simulink model "LSM_with_Simulek_CLM"  (R2016a)
settings: Solver=VariableStepAuto  StartTime=0.0  StopTime=2  RelTol=1e-3
values from neighbouring files (symbols this model uses):
  Theta = inv(R'*R)*R'*Y    [LSM with n=0 _ 1_1023 + 1105.m]    (also in LSM with n=2 _ more_1105.m = inv(R'*R)*R'* (Y2'); LSM_with_Simulek_1218.m = inv(X2'*X2)*X2'*Fs)
  Theta_c = inv(X2'*X2)*X2'*Fs    [Constrained_Least_Square_Method_CLM_1218.m]
undefined symbols (not defined in the file or in its folder): g, ks, kv, m
libraries: simulink x1
settings Model: Creator=lg079127  LastModifiedBy=lg079127

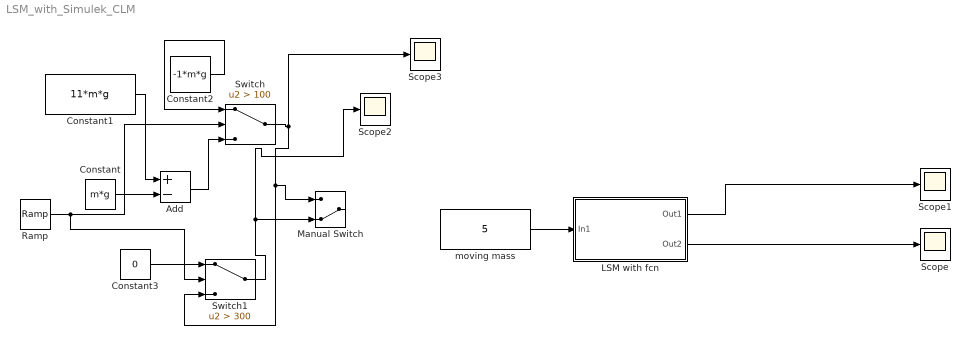
== system LSM_with_Simulek_CLM ==
  Add : Sum  Inputs=+-
  Constant : Constant  Value=m*g
  Constant1 : Constant  Value=11*m*g
  Constant2 : Constant  Value=-1*m*g
  Constant3 : Constant  Value=0
  LSM with fcn : Subsystem
  Manual Switch : ManualSwitch  CurrentSetting=0
  Ramp : simulink/Sources/Ramp  slope=1  start=0  X0=0
  Scope{,1..3} (4 alike) : Scope
  Switch : Switch  Criteria=u2 > Threshold  Threshold=100
  Switch1 : Switch  Criteria=u2 > Threshold  Threshold=300
  moving mass : Constant  Value=5
  wires:
  Switch/1 -> Scope3/1, Manual Switch/1, Switch1/3
  Constant1/1 -> Add/1
  Constant/1 -> Add/2
  Add/1 -> Switch/3
  Constant2/1 -> Switch/1
  Ramp/1 -> Switch1/2, Switch/2
  Constant3/1 -> Switch1/1
  Switch1/1 -> Manual Switch/2, Scope2/1
  LSM with fcn/1(Out1) -> Scope1/1
  LSM with fcn/2(Out2) -> Scope/1
  moving mass/1 -> LSM with fcn/1(In1)

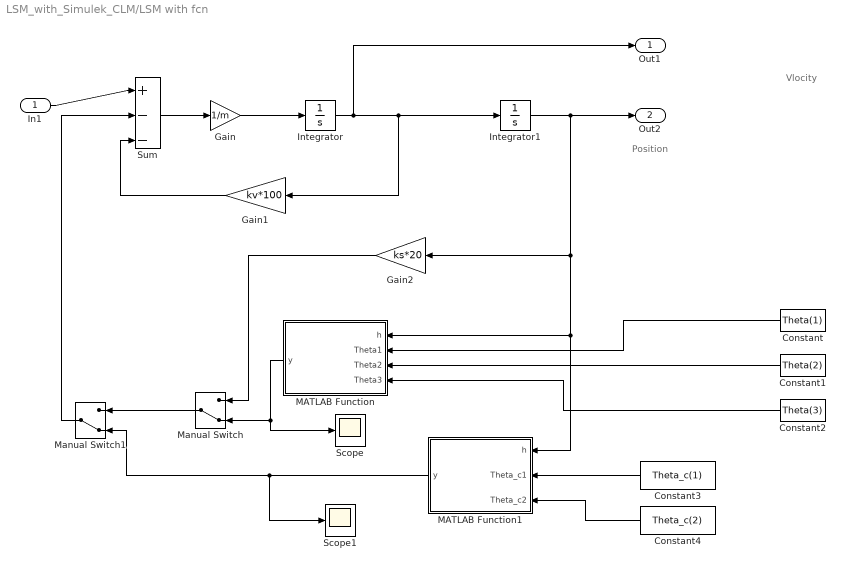
== system LSM_with_Simulek_CLM/LSM with fcn ==
  note: Position
  note: Vlocity
  In1 : Inport
  Constant : Constant  Value=Theta(1)
  Constant1 : Constant  Value=Theta(2)
  Constant2 : Constant  Value=Theta(3)
  Constant3 : Constant  Value=Theta_c(1)
  Constant4 : Constant  Value=Theta_c(2)
  Gain : Gain  Gain=1/m
  Gain1 : Gain  Gain=kv*100
  Gain2 : Gain  Gain=ks*20
  Integrator : Integrator
  Integrator1 : Integrator
  MATLAB Function : MATLAB Function  TreatAsAtomicUnit=on
  MATLAB Function1 : MATLAB Function  TreatAsAtomicUnit=on
  Manual Switch : ManualSwitch  CurrentSetting=0
  Manual Switch1 : ManualSwitch  CurrentSetting=0
  Scope : Scope
  Scope1 : Scope
  Sum : Sum  Inputs=|+--
  Out1 : Outport
  Out2 : Outport  Port=2
  wires:
  In1/1 -> Sum/1
  Sum/1 -> Gain/1
  Integrator/1 -> Out1/1, Gain1/1, Integrator1/1
  Gain/1 -> Integrator/1
  Gain1/1 -> Sum/3
  Manual Switch1/1 -> Sum/2
  Constant/1 -> MATLAB Function/2(Theta1)
  Constant1/1 -> MATLAB Function/3(Theta2)
  Constant2/1 -> MATLAB Function/4(Theta3)
  MATLAB Function/1(y) -> Scope/1, Manual Switch/2
  Gain2/1 -> Manual Switch/1
  Constant3/1 -> MATLAB Function1/2(Theta_c1)
  Constant4/1 -> MATLAB Function1/3(Theta_c2)
  Manual Switch/1 -> Manual Switch1/1
  MATLAB Function1/1(y) -> Scope1/1, Manual Switch1/2
  Integrator1/1 -> MATLAB Function1/1(h), MATLAB Function/1(h), Gain2/1, Out2/1

== matlab function LSM_with_Simulek_CLM/LSM with fcn/MATLAB Function1 ==
  data: h input; y output; Theta_c1 input; Theta_c2 input
function y = fcn(h,Theta_c1,Theta_c2)

h=Theta_c1*h^2+Theta_c2*h;

y = h;

%Constrained Least Squared Method

== matlab function LSM_with_Simulek_CLM/LSM with fcn/MATLAB Function ==
  data: h input; y output; Theta1 input; Theta2 input; Theta3 input
function y = fcn(h,Theta1,Theta2,Theta3)

h=Theta1*h^2+Theta2*h+Theta3;

y = h;
